simulink model "FullRate_BB_CDR"  (R2012b)
settings: Solver=ode45  StartTime=0.0  StopTime=10000/fbit  RelTol=1e-3
values from neighbouring files (symbols this model uses):
  fbit = 1    [init_pr_bb_cdr.m]
  OSR = 100    [init_pr_bb_cdr.m]
  PI_values = PI_values(1:end-1)    [init_pr_bb_cdr.m]
  ppm = 0    [init_pr_bb_cdr.m]
  SJ_amp = 0.3    [init_pr_bb_cdr.m]
  SJ_freq = fbit/1000    (= 0.001)    [init_pr_bb_cdr.m]
  Ts = 1/fbit/OSR    (= 0.01)    [init_pr_bb_cdr.m]
libraries: simulink_extras x10
settings Model: Creator=Tony  LastModifiedBy=Tony

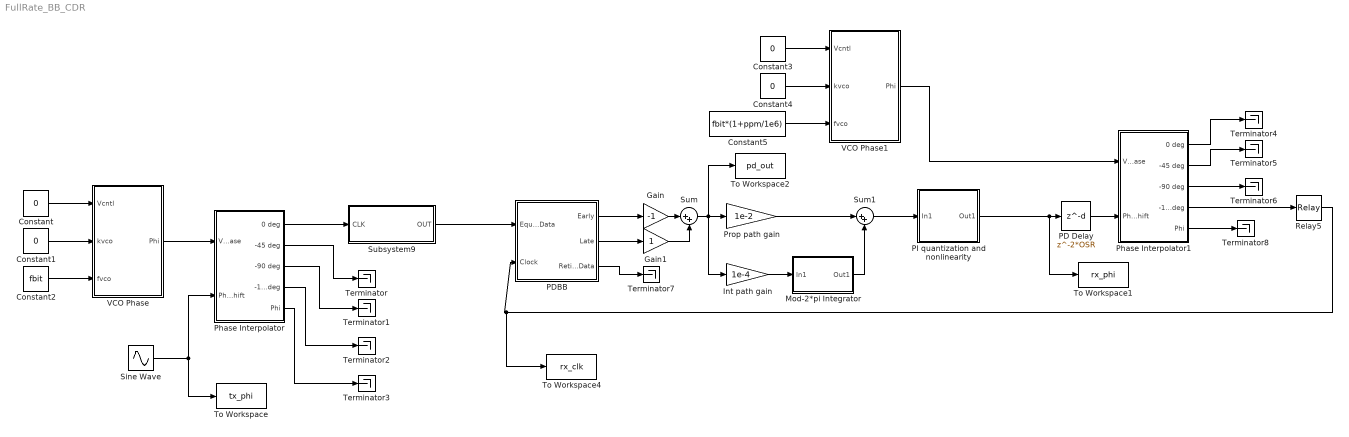
== system FullRate_BB_CDR ==
  Constant{,1,3..4} (4 alike) : Constant  Value=0
  Constant2 : Constant  Value=fbit
  Constant5 : Constant  Value=fbit*(1+ppm/1e6)
  Gain : Gain  Gain=-1
  Gain1 : Gain
  Int path gain : Gain  Gain=1e-4
  Mod-2*pi Integrator : Subsystem
  PD Delay : Delay  DelayLength=2*OSR
  PDBB : Subsystem  mask{VDD=1}
  PI quantization and nonlinearity : Subsystem
  Phase Interpolator : Subsystem  mask(Quad VCO){Ts=Ts}
      mask prompts: Ts "Sampling Time"
  Phase Interpolator1 : Subsystem  mask(Quad VCO){Ts=Ts}
      mask prompts: Ts "Sampling Time"
  Prop path gain : Gain  Gain=1e-2
  Relay5 : Relay  OffSwitchValue=-eps  OutDataTypeStr=Inherit: Inherit via back propagation
  Sine Wave : Sin  Amplitude=2*pi*SJ_amp  Frequency=SJ_freq  SampleTime=Ts
  Subsystem9 : Subsystem  mask{rst_time=100*Ts, X00=1, X01=1, X02=1, X03=1, X04=1, X05=1, X06=1, X07=1, X08=1, X09=1}
      mask prompts: rst_time "Reset time"; X00 "X00 [0,1]:"; X01 "X01 [0,1]:"; X02 "X02 [0,1]:"; X03 "X03 [0,1]:"; X04 "X04 [0,1]:"; X05 "X05 [0,1]:"; X06 "X06 [0,1]:"; X07 "X07 [0,1]:"; X08 "X08 [0,1]:"; X09 "X09 [0,1]:"
      mask help: Enter the initial state [0,1] below.
      mask Display: disp('PRBS_2^10')
  Sum : Sum  Inputs=|++
  Sum1 : Sum  Inputs=|++
  Terminator{,1..8} (9 alike) : Terminator
  To Workspace : ToWorkspace  VariableName=tx_phi  SampleTime=-1
  To Workspace1 : ToWorkspace  VariableName=rx_phi  SampleTime=-1
  To Workspace2 : ToWorkspace  VariableName=pd_out  SampleTime=-1
  To Workspace4 : ToWorkspace  VariableName=rx_clk  SampleTime=-1
  VCO Phase : Subsystem  mask(Quad VCO){po=0, center=0, Ts=Ts}
      mask prompts: po "Initial Phase (degrees)"; center "Voltage for Free-Running Freq"; Ts "Sampling Time"
      mask init:
      | ph_init = (po/360)*2*pi;
  VCO Phase1 : Subsystem  mask(Quad VCO){po=0, center=0, Ts=Ts}
      mask prompts: po "Initial Phase (degrees)"; center "Voltage for Free-Running Freq"; Ts "Sampling Time"
      mask init:
      | ph_init = (po/360)*2*pi;
  wires:
  Sine Wave/1 -> To Workspace/1, Phase Interpolator/2(Phase Shift)
  Constant/1 -> VCO Phase/1(Vcntl)
  Constant1/1 -> VCO Phase/2(kvco)
  Constant2/1 -> VCO Phase/3(fvco)
  Phase Interpolator/1(0 deg) -> Subsystem9/1(CLK)
  Phase Interpolator/2(-45 deg) -> Terminator/1
  Phase Interpolator/3(-90 deg) -> Terminator1/1
  Phase Interpolator/4(-135 deg) -> Terminator2/1
  Phase Interpolator/5(Phi) -> Terminator3/1
  Subsystem9/1(OUT) -> PDBB/1(EqualizedData)
  VCO Phase/1(Phi) -> Phase Interpolator/1(VCO Phase)
  Constant3/1 -> VCO Phase1/1(Vcntl)
  Constant4/1 -> VCO Phase1/2(kvco)
  Constant5/1 -> VCO Phase1/3(fvco)
  VCO Phase1/1(Phi) -> Phase Interpolator1/1(VCO Phase)
  Gain/1 -> Sum/1
  Gain1/1 -> Sum/2
  PDBB/1(Early) -> Gain/1
  PDBB/2(Late) -> Gain1/1
  Sum/1 -> To Workspace2/1, Int path gain/1, Prop path gain/1
  Int path gain/1 -> Mod-2*pi Integrator/1(In1)
  Prop path gain/1 -> Sum1/1
  Mod-2*pi Integrator/1(Out1) -> Sum1/2
  Phase Interpolator1/1(0 deg) -> Terminator4/1
  Phase Interpolator1/2(-45 deg) -> Terminator5/1
  Phase Interpolator1/3(-90 deg) -> Terminator6/1
  Phase Interpolator1/4(-135 deg) -> Relay5/1
  Relay5/1 -> To Workspace4/1, PDBB/2(Clock)
  PDBB/3(RetimedData) -> Terminator7/1
  Phase Interpolator1/5(Phi) -> Terminator8/1
  PD Delay/1 -> Phase Interpolator1/2(Phase Shift)
  PI quantization and nonlinearity/1(Out1) -> To Workspace1/1, PD Delay/1
  Sum1/1 -> PI quantization and nonlinearity/1(In1)

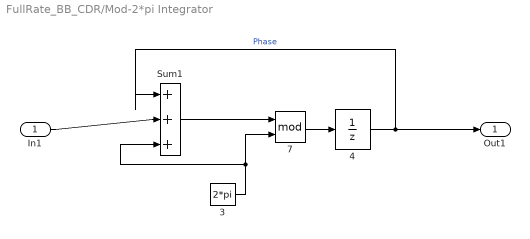
== system FullRate_BB_CDR/Mod-2*pi Integrator ==
  In1 : Inport
  3 : Constant  Value=2*pi
  4 : UnitDelay  SampleTime=Ts
  7 : Math  Operator=mod  SaturateOnIntegerOverflow=on
  Sum1 : Sum  Inputs=|+++  SaturateOnIntegerOverflow=on  InputSameDT=on  OutDataTypeStr=Inherit: Same as first input
  Out1 : Outport
  wires:
  7/1 -> 4/1
  3/1 -> Sum1/3, 7/2
  4/1 -> Out1/1, Sum1/1  "Phase"
  In1/1 -> Sum1/2
  Sum1/1 -> 7/1

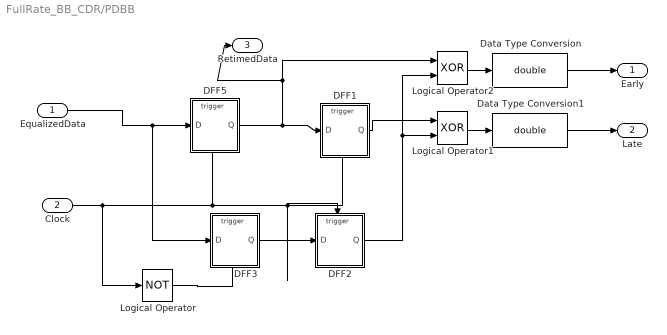
== system FullRate_BB_CDR/PDBB ==
  EqualizedData : Inport
  Clock : Inport  Port=2
  DFF1 : Subsystem  mask{DataHigh=VDD, DataLow=0, FF_Threshold=VDD/2}
      mask prompts: DataHigh "High Data Value"; DataLow "Low Data Value"; FF_Threshold "Flip-Flop Threshold"
  DFF2 : Subsystem  mask{DataHigh=VDD, DataLow=0, FF_Threshold=VDD/2}
      mask prompts: DataHigh "High Data Value"; DataLow "Low Data Value"; FF_Threshold "Flip-Flop Threshold"
  DFF3 : Subsystem  mask{DataHigh=VDD, DataLow=0, FF_Threshold=VDD/2}
      mask prompts: DataHigh "High Data Value"; DataLow "Low Data Value"; FF_Threshold "Flip-Flop Threshold"
  DFF5 : Subsystem  mask{DataHigh=VDD, DataLow=0, FF_Threshold=VDD/2}
      mask prompts: DataHigh "High Data Value"; DataLow "Low Data Value"; FF_Threshold "Flip-Flop Threshold"
  Data Type Conversion : DataTypeConversion  OutDataTypeStr=double
  Data Type Conversion1 : DataTypeConversion  OutDataTypeStr=double
  Logical Operator : Logic  Operator=NOT  AllPortsSameDT=off
  Logical Operator1 : Logic  Operator=XOR  AllPortsSameDT=off
  Logical Operator2 : Logic  Operator=XOR  AllPortsSameDT=off
  Early : Outport
  Late : Outport  Port=2
  RetimedData : Outport  Port=3
  wires:
  Clock/1 -> DFF2/Trigger, DFF1/Trigger, DFF5/Trigger, Logical Operator/1
  EqualizedData/1 -> DFF3/1(D), DFF5/1(D)
  Data Type Conversion1/1 -> Late/1
  Logical Operator1/1 -> Data Type Conversion1/1
  Data Type Conversion/1 -> Early/1
  Logical Operator2/1 -> Data Type Conversion/1
  Logical Operator/1 -> DFF3/Trigger
  DFF1/1(Q) -> Logical Operator1/1
  DFF2/1(Q) -> Logical Operator2/2, Logical Operator1/2
  DFF5/1(Q) -> DFF1/1(D), RetimedData/1, Logical Operator2/1
  DFF3/1(Q) -> DFF2/1(D)

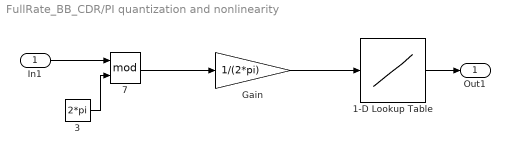
== system FullRate_BB_CDR/PI quantization and nonlinearity ==
  In1 : Inport
  1-D Lookup Table : Lookup_n-D  NumberOfTableDimensions=1  BreakpointsForDimension1=linspace(0,1-1/length(PI_values),length(PI_values))  Table=PI_values  InterpMethod=Flat  RndMeth=Simplest  InputSameDT=on
  3 : Constant  Value=2*pi
  7 : Math  Operator=mod  SaturateOnIntegerOverflow=on
  Gain : Gain  Gain=1/(2*pi)
  Out1 : Outport
  wires:
  Gain/1 -> 1-D Lookup Table/1
  7/1 -> Gain/1
  In1/1 -> 7/1
  3/1 -> 7/2
  1-D Lookup Table/1 -> Out1/1

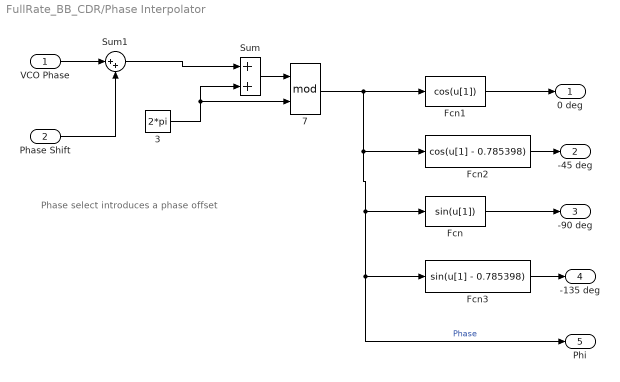
== system FullRate_BB_CDR/Phase Interpolator ==
  note: Phase select introduces a phase offset
  VCO Phase : Inport
  Phase Shift : Inport  Port=2
  3 : Constant  Value=2*pi
  7 : Math  Operator=mod  SaturateOnIntegerOverflow=on
  Fcn : Fcn  SampleTime=Ts
  Fcn1 : Fcn  Expr=cos(u[1])  SampleTime=Ts
  Fcn2 : Fcn  Expr=cos(u[1] - 0.785398)  SampleTime=Ts
  Fcn3 : Fcn  Expr=sin(u[1] - 0.785398)  SampleTime=Ts
  Sum : Sum  SaturateOnIntegerOverflow=on  InputSameDT=on  OutDataTypeStr=Inherit: Same as first input
  Sum1 : Sum  Inputs=|++  SaturateOnIntegerOverflow=on  InputSameDT=on  OutDataTypeStr=Inherit: Same as first input
  0 deg : Outport
  -45 deg : Outport  Port=2
  -90 deg : Outport  Port=3
  -135 deg : Outport  Port=4
  Phi : Outport  Port=5
  wires:
  Sum1/1 -> Sum/1
  Fcn3/1 -> -135 deg/1
  Fcn2/1 -> -45 deg/1
  3/1 -> 7/2, Sum/2
  Fcn1/1 -> 0 deg/1
  Fcn/1 -> -90 deg/1
  VCO Phase/1 -> Sum1/1
  Phase Shift/1 -> Sum1/2
  Sum/1 -> 7/1
  7/1 -> Phi/1, Fcn3/1, Fcn/1, Fcn2/1, Fcn1/1  "Phase"

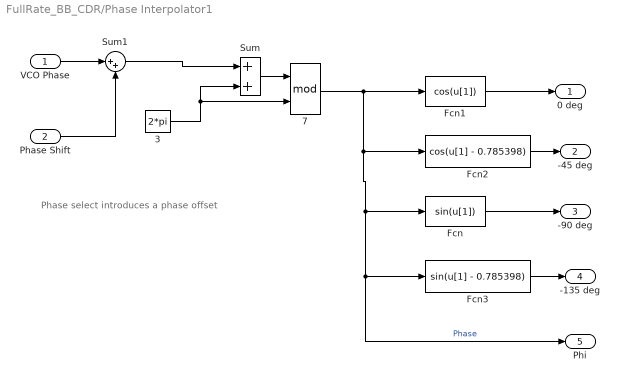
== system FullRate_BB_CDR/Phase Interpolator1 ==
  note: Phase select introduces a phase offset
  VCO Phase : Inport
  Phase Shift : Inport  Port=2
  3 : Constant  Value=2*pi
  7 : Math  Operator=mod  SaturateOnIntegerOverflow=on
  Fcn : Fcn  SampleTime=Ts
  Fcn1 : Fcn  Expr=cos(u[1])  SampleTime=Ts
  Fcn2 : Fcn  Expr=cos(u[1] - 0.785398)  SampleTime=Ts
  Fcn3 : Fcn  Expr=sin(u[1] - 0.785398)  SampleTime=Ts
  Sum : Sum  SaturateOnIntegerOverflow=on  InputSameDT=on  OutDataTypeStr=Inherit: Same as first input
  Sum1 : Sum  Inputs=|++  SaturateOnIntegerOverflow=on  InputSameDT=on  OutDataTypeStr=Inherit: Same as first input
  0 deg : Outport
  -45 deg : Outport  Port=2
  -90 deg : Outport  Port=3
  -135 deg : Outport  Port=4
  Phi : Outport  Port=5
  wires:
  7/1 -> Fcn1/1, Fcn2/1, Fcn/1, Fcn3/1, Phi/1  "Phase"
  Sum/1 -> 7/1
  Phase Shift/1 -> Sum1/2
  VCO Phase/1 -> Sum1/1
  Fcn/1 -> -90 deg/1
  Fcn1/1 -> 0 deg/1
  3/1 -> Sum/2, 7/2
  Fcn2/1 -> -45 deg/1
  Fcn3/1 -> -135 deg/1
  Sum1/1 -> Sum/1

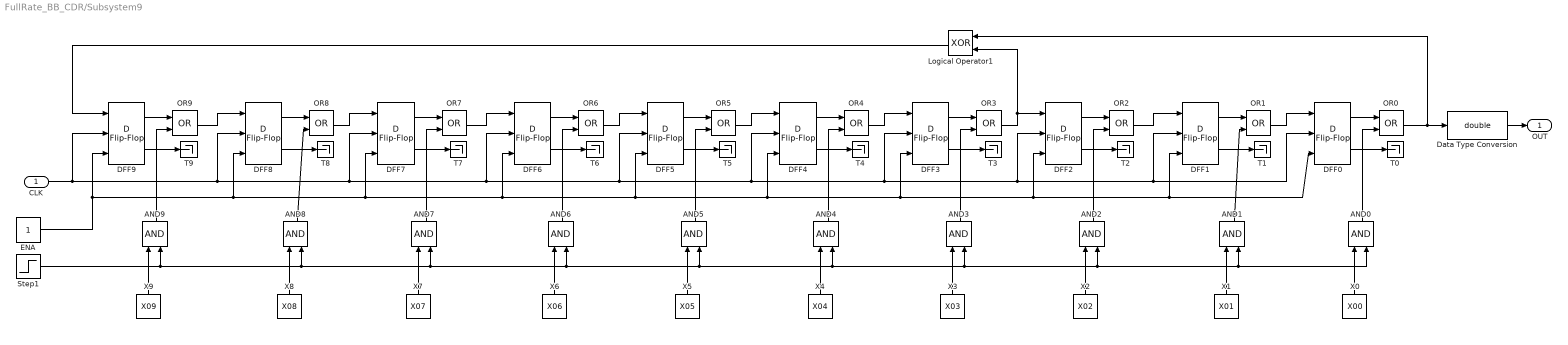
== system FullRate_BB_CDR/Subsystem9 ==
  CLK : Inport
  AND{0..9} (10 alike) : Logic  AllPortsSameDT=off  OutDataTypeStr=boolean
  DFF{0..9} (10 alike) : simulink_extras/Flip Flops/D Flip-Flop
  Data Type Conversion : DataTypeConversion  OutDataTypeStr=double
  ENA : Constant  OutDataTypeStr=boolean  SampleTime=-1
  Logical Operator1 : Logic  Operator=XOR  AllPortsSameDT=off  OutDataTypeStr=boolean
  OR{0..9} (10 alike) : Logic  Operator=OR  AllPortsSameDT=off  OutDataTypeStr=boolean
  Step1 : Step  Time=rst_time  Before=1  After=0
  T{0..9} (10 alike) : Terminator
  X0 : Constant  Value=X00  OutDataTypeStr=boolean  SampleTime=-1
  X1 : Constant  Value=X01  OutDataTypeStr=boolean  SampleTime=-1
  X2 : Constant  Value=X02  OutDataTypeStr=boolean  SampleTime=-1
  X3 : Constant  Value=X03  OutDataTypeStr=boolean  SampleTime=-1
  X4 : Constant  Value=X04  OutDataTypeStr=boolean  SampleTime=-1
  X5 : Constant  Value=X05  OutDataTypeStr=boolean  SampleTime=-1
  X6 : Constant  Value=X06  OutDataTypeStr=boolean  SampleTime=-1
  X7 : Constant  Value=X07  OutDataTypeStr=boolean  SampleTime=-1
  X8 : Constant  Value=X08  OutDataTypeStr=boolean  SampleTime=-1
  X9 : Constant  Value=X09  OutDataTypeStr=boolean  SampleTime=-1
  OUT : Outport
  wires:
  Data Type Conversion/1 -> OUT/1
  Step1/1 -> AND6/2, AND4/2, AND3/2, AND2/2, AND1/2, AND0/2, AND5/2, AND7/2, AND8/2, AND9/2
  Logical Operator1/1 -> DFF9/1
  ENA/1 -> DFF5/3, DFF3/3, DFF2/3, DFF1/3, DFF0/3, DFF4/3, DFF6/3, DFF7/3, DFF8/3, DFF9/3
  CLK/1 -> DFF4/2, DFF3/2, DFF2/2, DFF1/2, DFF0/2, DFF5/2, DFF6/2, DFF7/2, DFF8/2, DFF9/2
  OR7/1 -> DFF6/1
  X9/1 -> AND9/1
  X7/1 -> AND7/1
  X8/1 -> AND8/1
  DFF9/1 -> OR9/1
  DFF9/2 -> T9/1
  DFF8/1 -> OR8/1
  DFF8/2 -> T8/1
  OR9/1 -> DFF8/1
  DFF7/1 -> OR7/1
  DFF7/2 -> T7/1
  OR8/1 -> DFF7/1
  AND8/1 -> OR8/2
  AND7/1 -> OR7/2
  AND9/1 -> OR9/2
  X2/1 -> AND2/1
  X0/1 -> AND0/1
  X5/1 -> AND5/1
  X4/1 -> AND4/1
  X3/1 -> AND3/1
  X1/1 -> AND1/1
  X6/1 -> AND6/1
  DFF6/1 -> OR6/1
  DFF6/2 -> T6/1
  DFF5/1 -> OR5/1
  DFF5/2 -> T5/1
  OR6/1 -> DFF5/1
  DFF4/1 -> OR4/1
  DFF4/2 -> T4/1
  OR5/1 -> DFF4/1
  DFF3/1 -> OR3/1
  DFF3/2 -> T3/1
  OR4/1 -> DFF3/1
  DFF2/1 -> OR2/1
  DFF2/2 -> T2/1
  OR3/1 -> Logical Operator1/2, DFF2/1
  DFF1/1 -> OR1/1
  DFF1/2 -> T1/1
  OR2/1 -> DFF1/1
  DFF0/1 -> OR0/1
  DFF0/2 -> T0/1
  OR1/1 -> DFF0/1
  OR0/1 -> Data Type Conversion/1, Logical Operator1/1
  AND1/1 -> OR1/2
  AND0/1 -> OR0/2
  AND2/1 -> OR2/2
  AND3/1 -> OR3/2
  AND4/1 -> OR4/2
  AND5/1 -> OR5/2
  AND6/1 -> OR6/2

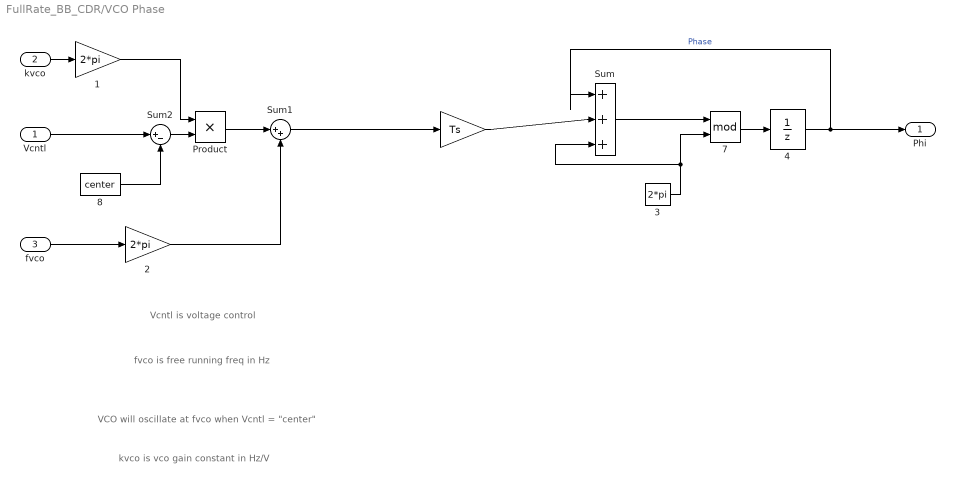
== system FullRate_BB_CDR/VCO Phase ==
  note: fvco is free running
      | freq in Hz
  note: kvco is vco gain
      | constant in Hz/V
  note: Vcntl is voltage control
  note: VCO will oscillate at fvco
      | when Vcntl = "center"
  Vcntl : Inport
  kvco : Inport  Port=2
  fvco : Inport  Port=3
  " " : Gain  Gain=Ts  SaturateOnIntegerOverflow=on  OutDataTypeStr=Inherit: Same as input  ParamDataTypeStr=Inherit: Same as input
  " 1" : Gain  Gain=2*pi  SaturateOnIntegerOverflow=on  OutDataTypeStr=Inherit: Same as input  ParamDataTypeStr=Inherit: Same as input
  " 2" : Gain  Gain=2*pi  SaturateOnIntegerOverflow=on  OutDataTypeStr=Inherit: Same as input  ParamDataTypeStr=Inherit: Same as input
  3 : Constant  Value=2*pi
  4 : UnitDelay  InitialCondition=ph_init  SampleTime=Ts
  7 : Math  Operator=mod  SaturateOnIntegerOverflow=on
  8 : Constant  Value=center
  Product : Product  SaturateOnIntegerOverflow=on  InputSameDT=on  OutDataTypeStr=Inherit: Same as first input
  Sum : Sum  Inputs=|+++  SaturateOnIntegerOverflow=on  InputSameDT=on  OutDataTypeStr=Inherit: Same as first input
  Sum1 : Sum  Inputs=|++  SaturateOnIntegerOverflow=on  InputSameDT=on  OutDataTypeStr=Inherit: Same as first input
  Sum2 : Sum  Inputs=|+-  SaturateOnIntegerOverflow=on  InputSameDT=on  OutDataTypeStr=Inherit: Same as first input
  Phi : Outport
  wires:
  3/1 -> Sum/3, 7/2
  Product/1 -> Sum1/1
  " 1"/1 -> Product/1
  kvco/1 -> " 1"/1
  fvco/1 -> " 2"/1
  " 2"/1 -> Sum1/2
  Sum2/1 -> Product/2
  Vcntl/1 -> Sum2/1
  8/1 -> Sum2/2
  " "/1 -> Sum/2
  Sum/1 -> 7/1
  Sum1/1 -> " "/1
  7/1 -> 4/1
  4/1 -> Phi/1, Sum/1  "Phase"

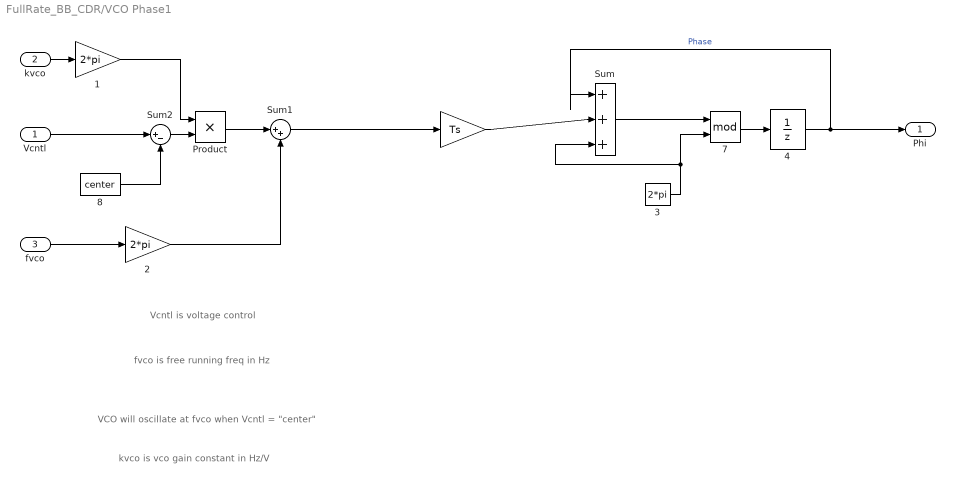
== system FullRate_BB_CDR/VCO Phase1 ==
  note: VCO will oscillate at fvco
      | when Vcntl = "center"
  note: Vcntl is voltage control
  note: kvco is vco gain
      | constant in Hz/V
  note: fvco is free running
      | freq in Hz
  Vcntl : Inport
  kvco : Inport  Port=2
  fvco : Inport  Port=3
  " " : Gain  Gain=Ts  SaturateOnIntegerOverflow=on  OutDataTypeStr=Inherit: Same as input  ParamDataTypeStr=Inherit: Same as input
  " 1" : Gain  Gain=2*pi  SaturateOnIntegerOverflow=on  OutDataTypeStr=Inherit: Same as input  ParamDataTypeStr=Inherit: Same as input
  " 2" : Gain  Gain=2*pi  SaturateOnIntegerOverflow=on  OutDataTypeStr=Inherit: Same as input  ParamDataTypeStr=Inherit: Same as input
  3 : Constant  Value=2*pi
  4 : UnitDelay  InitialCondition=ph_init  SampleTime=Ts
  7 : Math  Operator=mod  SaturateOnIntegerOverflow=on
  8 : Constant  Value=center
  Product : Product  SaturateOnIntegerOverflow=on  InputSameDT=on  OutDataTypeStr=Inherit: Same as first input
  Sum : Sum  Inputs=|+++  SaturateOnIntegerOverflow=on  InputSameDT=on  OutDataTypeStr=Inherit: Same as first input
  Sum1 : Sum  Inputs=|++  SaturateOnIntegerOverflow=on  InputSameDT=on  OutDataTypeStr=Inherit: Same as first input
  Sum2 : Sum  Inputs=|+-  SaturateOnIntegerOverflow=on  InputSameDT=on  OutDataTypeStr=Inherit: Same as first input
  Phi : Outport
  wires:
  4/1 -> Sum/1, Phi/1  "Phase"
  7/1 -> 4/1
  Sum1/1 -> " "/1
  Sum/1 -> 7/1
  " "/1 -> Sum/2
  8/1 -> Sum2/2
  Vcntl/1 -> Sum2/1
  Sum2/1 -> Product/2
  " 2"/1 -> Sum1/2
  fvco/1 -> " 2"/1
  kvco/1 -> " 1"/1
  " 1"/1 -> Product/1
  Product/1 -> Sum1/1
  3/1 -> 7/2, Sum/3

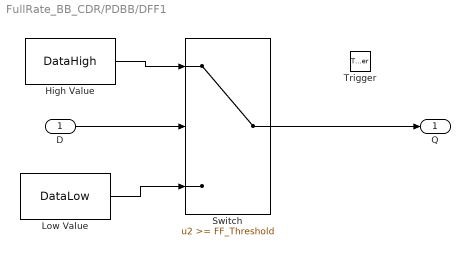
== system FullRate_BB_CDR/PDBB/DFF1 ==
  D : Inport  LatchByDelayingOutsideSignal=on
  Trigger : TriggerPort
  High Value : Constant  Value=DataHigh
  Low Value : Constant  Value=DataLow
  Switch : Switch  Threshold=FF_Threshold
  Q : Outport
  wires:
  Low Value/1 -> Switch/3
  High Value/1 -> Switch/1
  D/1 -> Switch/2
  Switch/1 -> Q/1

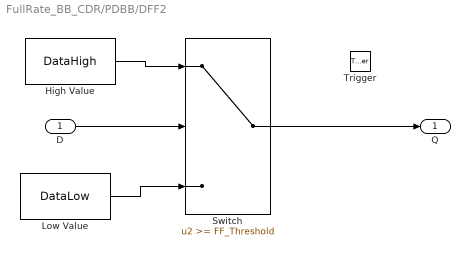
== system FullRate_BB_CDR/PDBB/DFF2 ==
  D : Inport  LatchByDelayingOutsideSignal=on
  Trigger : TriggerPort
  High Value : Constant  Value=DataHigh
  Low Value : Constant  Value=DataLow
  Switch : Switch  Threshold=FF_Threshold
  Q : Outport
  wires:
  Low Value/1 -> Switch/3
  High Value/1 -> Switch/1
  D/1 -> Switch/2
  Switch/1 -> Q/1

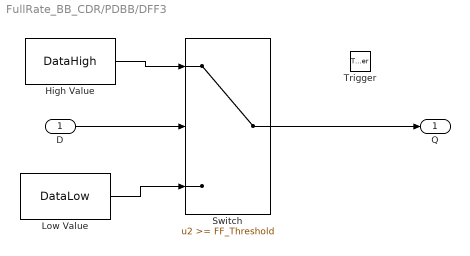
== system FullRate_BB_CDR/PDBB/DFF3 ==
  D : Inport  LatchByDelayingOutsideSignal=on
  Trigger : TriggerPort
  High Value : Constant  Value=DataHigh
  Low Value : Constant  Value=DataLow
  Switch : Switch  Threshold=FF_Threshold
  Q : Outport
  wires:
  Low Value/1 -> Switch/3
  High Value/1 -> Switch/1
  D/1 -> Switch/2
  Switch/1 -> Q/1

== system FullRate_BB_CDR/PDBB/DFF5 ==
  D : Inport  LatchByDelayingOutsideSignal=on
  Trigger : TriggerPort
  High Value : Constant  Value=DataHigh
  Low Value : Constant  Value=DataLow
  Switch : Switch  Threshold=FF_Threshold
  Q : Outport
  wires:
  Low Value/1 -> Switch/3
  High Value/1 -> Switch/1
  D/1 -> Switch/2
  Switch/1 -> Q/1
